simulink model "ies_DCMotorControl"  (R2014a)
settings: Solver=ode45  StartTime=0.0  StopTime=8  RelTol=1e-3
values from neighbouring files (symbols this model uses):
  Kd = 10    [DCMotorControlSetup.mat]
  Ki = 200    [DCMotorControlSetup.mat]
  Kp = 100    [DCMotorControlSetup.mat]
  Ts = 0.05    [DCMotorControlSetup.mat]
settings Model: Creator=matteo  LastModifiedBy=matteo
settings DebuggingCC: SolverPrmCheckMsg=none

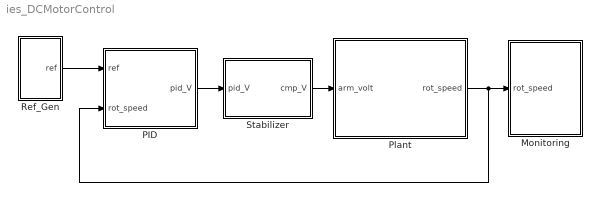
== system ies_DCMotorControl ==
  Monitoring : Subsystem  Tag=Monitoring
  PID : Subsystem  TreatAsAtomicUnit=on  SystemSampleTime=Ts
  Plant : Subsystem  Tag=Plant
  Ref_Gen : Subsystem  TreatAsAtomicUnit=on  SystemSampleTime=2*Ts
  Stabilizer : Subsystem  TreatAsAtomicUnit=on  SystemSampleTime=Ts
  wires:
  Plant/1(rot_speed) -> PID/2(rot_speed), Monitoring/1(rot_speed)
  Stabilizer/1(cmp_V) -> Plant/1(arm_volt)
  PID/1(pid_V) -> Stabilizer/1(pid_V)
  Ref_Gen/1(ref) -> PID/1(ref)

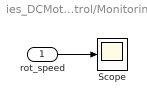
== system ies_DCMotorControl/Monitoring ==
  rot_speed : Inport
  Scope : Scope
  wires:
  rot_speed/1 -> Scope/1

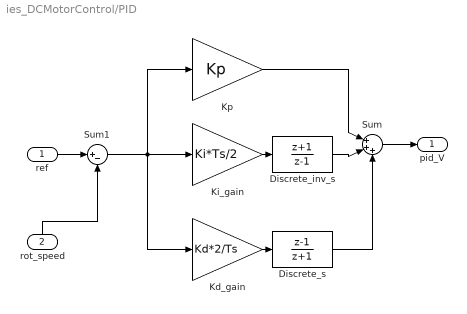
== system ies_DCMotorControl/PID ==
  ref : Inport
  rot_speed : Inport  Port=2
  Discrete_inv_s : DiscreteTransferFcn  DialogController=Simulink.DDGSource  Numerator=[1 1]  Denominator=[1 -1]
  Discrete_s : DiscreteTransferFcn  Numerator=[1 -1]  Denominator=[1 1]
  Kd_gain : Gain  Gain=Kd*2/Ts
  Ki_gain : Gain  Gain=Ki*Ts/2
  Kp : Gain  Gain=Kp
  Sum : Sum  Inputs=|+++
  Sum1 : Sum  Inputs=|+-
  pid_V : Outport
  wires:
  Sum1/1 -> Kd_gain/1, Ki_gain/1, Kp/1
  ref/1 -> Sum1/1
  Kd_gain/1 -> Discrete_s/1
  Sum/1 -> pid_V/1
  rot_speed/1 -> Sum1/2
  Ki_gain/1 -> Discrete_inv_s/1
  Discrete_s/1 -> Sum/3
  Kp/1 -> Sum/1
  Discrete_inv_s/1 -> Sum/2

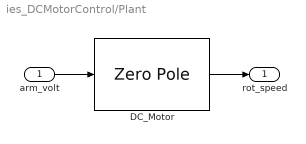
== system ies_DCMotorControl/Plant ==
  arm_volt : Inport  SampleTime=0
  DC_Motor : ZeroPole  Zeros=[]  Poles=[-9.9975 -2.0025]  Gain=[2]
  rot_speed : Outport
  wires:
  DC_Motor/1 -> rot_speed/1
  arm_volt/1 -> DC_Motor/1

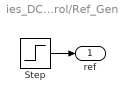
== system ies_DCMotorControl/Ref_Gen ==
  Step : Step
  ref : Outport
  wires:
  Step/1 -> ref/1

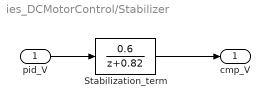
== system ies_DCMotorControl/Stabilizer ==
  pid_V : Inport
  Stabilization_term : DiscreteTransferFcn  Numerator=[0.6]  Denominator=[1 0.82]
  cmp_V : Outport
  wires:
  Stabilization_term/1 -> cmp_V/1
  pid_V/1 -> Stabilization_term/1
